simulink model "model_problem1"  (R2020a)
settings: Solver=VariableStepAuto  StartTime=0.0  StopTime=10  RelTol=1e-3
libraries: simulink_extras x1
settings Model: EnablePacing=on  Creator=Prateek  LastModifiedBy=Prateek

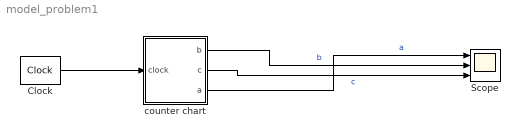
== system model_problem1 ==
  Clock : simulink_extras/Flip Flops/Clock  period=2
  Scope : Scope  NumInputPorts=3
  counter chart : Stateflow chart  TreatAsAtomicUnit=on
  wires:
  Clock/1 -> counter chart/1(clock)
  counter chart/3(a) -> Scope/1  "a"
  counter chart/1(b) -> Scope/2  "b"
  counter chart/2(c) -> Scope/3  "c"

== stateflow chart model_problem1/counter chart ==
  state state1
    entry:
    a=0;
    b=0;
    c=0;
  state state2
    entry:
    a=1;
    b=0;
    c=0;
  state state3
    entry:
    a=0;
    b=1;
    c=0;
  state state4
    entry:
    a=1;
    b=1;
    c=0;
  state state5
    entry:
    a=0;
    b=0;
    c=1;
  (default) -> state1
  state5 -> state1 : [c==1&&b==0&&a==0]
  state1 -> state2 : {c==0&& b==0&& a==0}
  state2 -> state3 : [c==0&&b==0&&a==1]
  state3 -> state4 : [c==0&&b==1&&a==0]
  state4 -> state5 : [c==0&&b==1&&a==1]
  data: clock input; b output; c output; a output
